simulink model "BirdHeadModel"  (R2023a)
settings: Solver=ode45  StartTime=0.0  StopTime=10.0  RelTol=1e-3
settings Model: Creator=coquet  LastModifiedBy=coquet

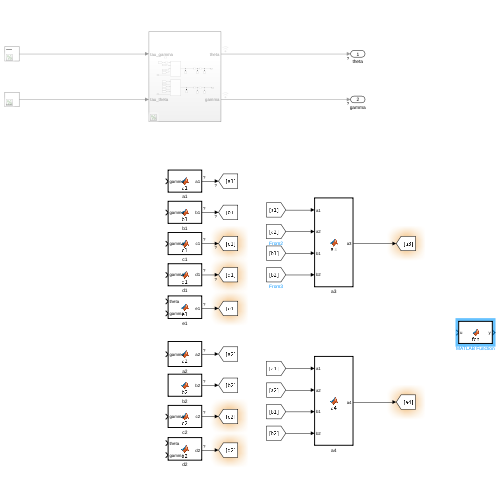
[thumbnail: Simulink's stored preview of the top-level diagram]
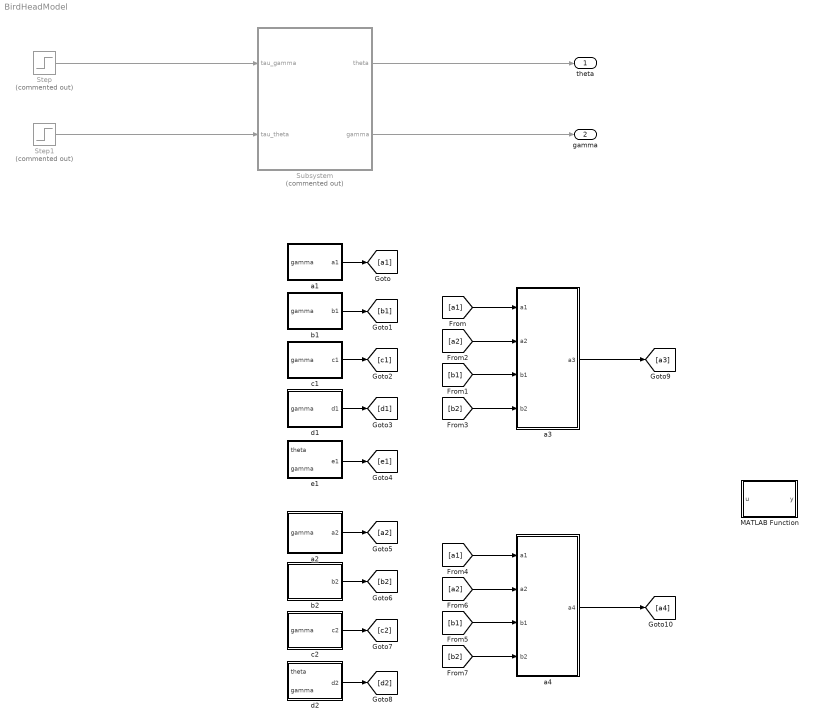
== system BirdHeadModel ==
  MATLAB Function : MATLAB Function  TreatAsAtomicUnit=on
  Step : Step  Commented=on  After=-1  SampleTime=0
  Step1 : Step  Commented=on  SampleTime=0
  Subsystem : Subsystem  Commented=on
  a1 : MATLAB Function  TreatAsAtomicUnit=on
  a2 : MATLAB Function  TreatAsAtomicUnit=on
  a3 : MATLAB Function  TreatAsAtomicUnit=on
  a4 : MATLAB Function  TreatAsAtomicUnit=on
  b1 : MATLAB Function  TreatAsAtomicUnit=on
  b2 : MATLAB Function  TreatAsAtomicUnit=on
  c1 : MATLAB Function  TreatAsAtomicUnit=on
  c2 : MATLAB Function  TreatAsAtomicUnit=on
  d1 : MATLAB Function  TreatAsAtomicUnit=on
  d2 : MATLAB Function  TreatAsAtomicUnit=on
  e1 : MATLAB Function  TreatAsAtomicUnit=on
  theta : Outport
  gamma : Outport  Port=2
  wires:
  Subsystem/1(theta) -> theta/1
  Subsystem/2(gamma) -> gamma/1
  Step/1 -> Subsystem/1(tau_gamma)
  Step1/1 -> Subsystem/2(tau_theta)
  a1/1(a1) -> [a1]
  b1/1(b1) -> [b1]
  c1/1(c1) -> [c1]
  d1/1(d1) -> [d1]
  e1/1(e1) -> [e1]
  a2/1(a2) -> [a2]
  b2/1(b2) -> [b2]
  c2/1(c2) -> [c2]
  d2/1(d2) -> [d2]
  [a1] -> a3/1(a1)
  [b1] -> a3/3(b1)
  [a2] -> a3/2(a2)
  [b2] -> a3/4(b2)
  [a1] -> a4/1(a1)
  [b1] -> a4/3(b1)
  [a2] -> a4/2(a2)
  [b2] -> a4/4(b2)
  a3/1(a3) -> [a3]
  a4/1(a4) -> [a4]

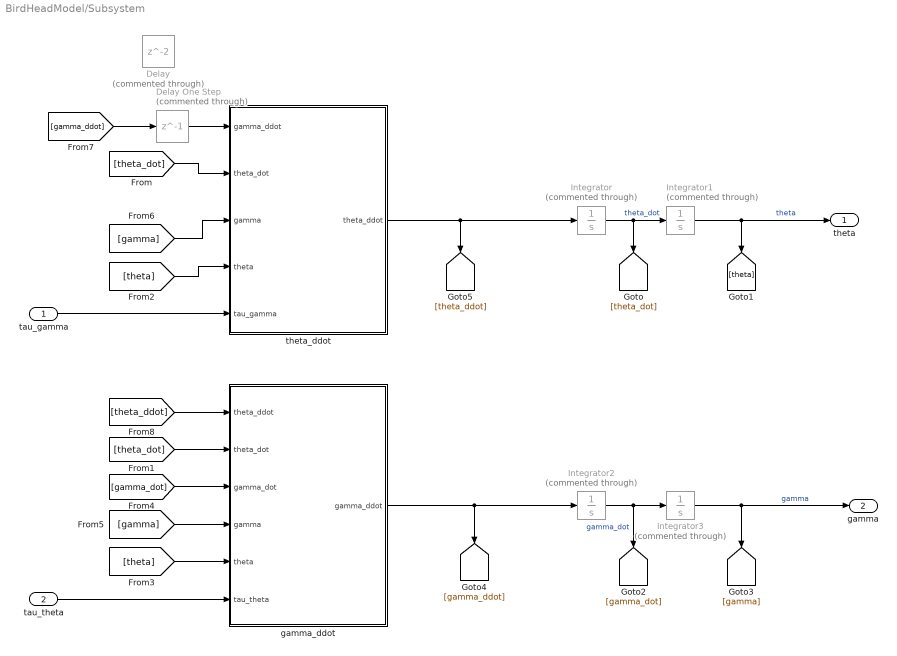
== system BirdHeadModel/Subsystem ==
  tau_gamma : Inport
  tau_theta : Inport  Port=2
  Delay : Delay  Commented=through
  Delay One Step : Delay  Commented=through  DelayLength=1
  Integrator : Integrator  Commented=through  ContinuousStateAttributes='theta_dot'
  Integrator1 : Integrator  Commented=through  UpperSaturationLimit=2*pi/9  LowerSaturationLimit=-pi/3  ContinuousStateAttributes='theta'
  Integrator2 : Integrator  Commented=through  ContinuousStateAttributes='gamma_dot'
  Integrator3 : Integrator  Commented=through  UpperSaturationLimit=2*pi/9  LowerSaturationLimit=-pi/3  ContinuousStateAttributes='gamma'
  gamma_ddot : MATLAB Function  TreatAsAtomicUnit=on
  theta_ddot : MATLAB Function  TreatAsAtomicUnit=on
  theta : Outport
  gamma : Outport  Port=2
  wires:
  [theta_dot] -> theta_ddot/2(theta_dot)
  tau_gamma/1 -> theta_ddot/5(tau_gamma)
  [gamma] -> theta_ddot/3(gamma)
  theta_ddot/1(theta_ddot) -> [theta_ddot], Integrator/1
  [gamma_dot] -> gamma_ddot/3(gamma_dot)
  [gamma] -> gamma_ddot/4(gamma)
  [theta_dot] -> gamma_ddot/2(theta_dot)
  [theta] -> theta_ddot/4(theta)
  [theta] -> gamma_ddot/5(theta)
  [theta_ddot] -> gamma_ddot/1(theta_ddot)
  tau_theta/1 -> gamma_ddot/6(tau_theta)
  Integrator2/1 -> [gamma_dot], Integrator3/1  "gamma_dot"
  Integrator1/1 -> theta/1, [theta]  "theta"
  gamma_ddot/1(gamma_ddot) -> Integrator2/1, [gamma_ddot]
  Integrator3/1 -> gamma/1, [gamma]  "gamma"
  Integrator/1 -> Integrator1/1, [theta_dot]  "theta_dot"
  Delay One Step/1 -> theta_ddot/1(gamma_ddot)
  [gamma_ddot] -> Delay One Step/1

== matlab function BirdHeadModel/a3 ==
  data: a1 input; a3 output; a2 input; b1 input; b2 input
function a3 = a3(a1,a2,b1,b2)

a3 = (b1/(a2*b1-a1*b2));

== matlab function BirdHeadModel/a4 ==
  data: a1 input; a4 output; a2 input; b1 input; b2 input
function a4 = a4(a1,a2,b1,b2)

a4 = (b2/(a2*b1-a1*b2));

== matlab function BirdHeadModel/MATLAB Function ==
  data: u input; y output
function y = fcn(u)

y = u;

== matlab function BirdHeadModel/Subsystem/gamma_ddot ==
  data: theta_ddot input; gamma_ddot output; theta_dot input; gamma_dot input; gamma input; theta input; tau_theta input
function gamma_ddot  = fcn(theta_ddot, theta_dot, gamma_dot, gamma, theta, tau_theta)
I_hy = 0.0001;
I_by = 0.0001;
l_h = 0.035;
l_b = 0.030;
m_h = 0.0049;
g = 9.8;

gamma_ddot = (tau_theta - ((I_hy+I_by+((l_b^2+l_h^2)*m_h+ 2*l_b*l_h*m_h*cos(gamma))*theta_ddot + (g*(l_h*m_h*sin(gamma - theta)-l_b*m_h*sin(theta))) + (2*l_h^2*m_h*cos(2*gamma) + l_b*l_h*m_h*cos(gamma))*gamma_dot^2 - 2*l_b*l_h *m_h*sin(gamma)*theta_dot*gamma_dot)))/(I_hy+l_h^2*m_h*sin(2*gamma)+l_b*l_h*m_h*sin(gamma));

== matlab function BirdHeadModel/Subsystem/theta_ddot ==
  data: gamma_ddot input; theta_ddot output; theta_dot input; gamma input; theta input; tau_gamma input
function theta_ddot  = fcn(gamma_ddot, theta_dot, gamma, theta, tau_gamma)
I_hy = 0.0001;
l_h = 0.035;
l_b = 0.030;
m_h = 0.0049;
g = 9.8;
theta_ddot = (tau_gamma - ((I_hy + l_h^2*m_h)*gamma_ddot + (g*l_h*m_h*cos(gamma + theta)) + l_b*l_h*m_h*sin(gamma)*theta_dot^2 ))/ (I_hy+l_h^2*m_h*sin(2*gamma) + l_b*l_h*m_h*sin(gamma));

== matlab function BirdHeadModel/a1 ==
  data: gamma input; a1 output
function a1 = a1(gamma)

a1 = I_hy+I_by+(l_b^2+l_h^2)*m_h+ 2*l_b*l_h*m_h*cos(gamma);

== matlab function BirdHeadModel/b1 ==
  data: gamma input; b1 output
function b1 = b1(gamma)

b1 = I_hy+l_h^2*m_h*sin(2*gamma)+l_b*l_h*m_h*sin(gamma);

== matlab function BirdHeadModel/c1 ==
  data: gamma input; c1 output
function c1 = c1(gamma)

c1 = 2*l_h^2*m_h*cos(2*gamma) + l_b*l_h*m_h*cos(gamma);

== matlab function BirdHeadModel/d1 ==
  data: gamma input; d1 output
function d1 = d1(gamma)

d1 = - 2*l_b*l_h *m_h*sin(gamma);

== matlab function BirdHeadModel/e1 ==
  data: theta input; gamma input; e1 output
function e1 = e1(theta, gamma)

e1 = l_h*m_h*sin(gamma - theta)-l_b*m_h*sin(theta);

== matlab function BirdHeadModel/a2 ==
  data: gamma input; a2 output
function a2 = a2(gamma)

a2 = I_hy+l_h^2*m_h*sin(2*gamma) + l_b*l_h*m_h*sin(gamma);

== matlab function BirdHeadModel/b2 ==
  data: b2 output
function b2 = b2()

b2 = I_hy + l_h^2*m_h;

== matlab function BirdHeadModel/c2 ==
  data: gamma input; c2 output
function c2 = c2(gamma)

c2 = l_b*l_h*m_h*sin(gamma);

== matlab function BirdHeadModel/d2 ==
  data: theta input; gamma input; d2 output
function d2 = d2(theta, gamma)

d2 = l_h*m_h*cos(gamma + theta);
